simulink model "trajectoryModel"  (Simulink 8.4)
settings: Solver=ode45  StartTime=0.0  StopTime=timeInterval(2)  FixedStep=1e-2  MaxStep=1e-3  RelTol=1e-4  AbsTol=1e-4
values from neighbouring files (symbols this model uses):
  closeRadius = 0.01657    [checkEscapeVelocity.m]
  initialConditions = [x, dx, y, dy]    [checkEscapeVelocity.m]
  mu = Moon_mass / M    (= 0.0121505482564)    [checkEscapeVelocity.m]    (also in computeJacobiCFromRAT.m; velocityPlot_script.m = 0)
  stopRadius = 2    [checkEscapeVelocity.m]
settings Model: Creator=eugene  LastModifiedBy=eugene
settings SolverCC: AutoInsertRateTranBlk=on
settings DataIOCC: SignalLoggingSaveFormat=Dataset
settings OptimizationCC: ExpressionDepthLimit=128  SimCompilerOptimization=On
settings DebuggingCC: UnderspecifiedInitializationDetection=Simplified  MergeDetectMultiDrivingBlocksExec=error  FcnCallInpInsideContextMsg=EnableAllAsError  StateNameClashWarn=none
settings GRTTargetCC: CombineOutputUpdateFcns=on  GRTInterface=off

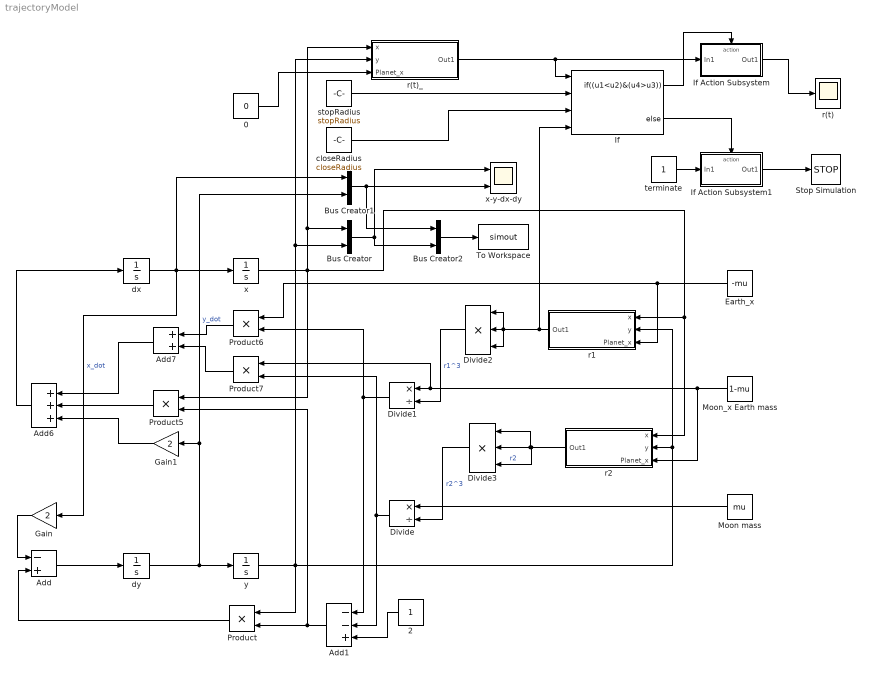
== system trajectoryModel ==
  "0 " : Constant  Value=0
  2 : Constant
  Add : Sum  Inputs=-+
  Add1 : Sum  Inputs=--+
  Add6 : Sum  Inputs=+++
  Add7 : Sum
  Bus Creator : BusCreator  Inputs=2
  Bus Creator1 : BusCreator  Inputs=2
  Bus Creator2 : BusCreator  Inputs=2
  Divide : Product  Inputs=*/
  Divide1 : Product  Inputs=*/
  Divide2 : Product  Inputs=***
  Divide3 : Product  Inputs=***
  Earth_x : Constant  Value=-mu
  Gain : Gain  Gain=2
  Gain1 : Gain  Gain=2
  If : If  NumInputs=4  IfExpression=(u1<u2)&(u4>u3)
  If Action Subsystem : Subsystem  TreatAsAtomicUnit=on
  If Action Subsystem1 : Subsystem  TreatAsAtomicUnit=on
  Moon mass : Constant  Value=mu
  Moon_x Earth mass : Constant  Value=1-mu
  Product{,5..7} (4 alike) : Product
  Stop Simulation : Stop
  To Workspace : ToWorkspace  VariableName=simout  SaveFormat=Timeseries  SampleTime=-1
  closeRadius : Constant  Value=closeRadius
  dx : Integrator  InitialCondition=initialConditions(2)  AbsoluteTolerance=1e-6
  dy : Integrator  InitialCondition=initialConditions(4)  AbsoluteTolerance=1e-6
  r(t) : Scope
      settings: ShowLegends=on  TimeRange=23
  r(t)_ : Subsystem
  r1 : Subsystem
  r2 : Subsystem
  stopRadius : Constant  Value=stopRadius
  terminate : Constant
  x : Integrator  InitialCondition=initialConditions(1)  AbsoluteTolerance=1e-6
  x-y-dx-dy : Scope  NumInputPorts=2
      settings: ShowLegends=on  TimeRange=23  YMin=-5~-5  YMax=5~5  SaveName=ScopeData3
  "y " : Integrator  InitialCondition=initialConditions(3)  AbsoluteTolerance=1e-6
  wires:
  dx/1 -> Bus Creator1/1, Gain/1, x/1  "x_dot"
  dy/1 -> Bus Creator1/2, Gain1/1, "y "/1  "y_dot"
  Earth_x/1 -> Product6/1, r1/3(Planet_x)
  Gain/1 -> Add/1
  Moon_x Earth mass/1 -> Divide1/1, Product7/1, r2/3(Planet_x)
  2/1 -> Add1/3
  Divide/1 -> Product7/2, Add1/2
  Divide1/1 -> Product6/2, Add1/1
  "y "/1 -> Product/1, r2/2(y), r1/2(y), r(t)_/2(y), Bus Creator/2
  Add1/1 -> Product5/2, Product/2
  Product/1 -> Add/2
  Add/1 -> dy/1
  x/1 -> r2/1(x), r1/1(x), Bus Creator/1, r(t)_/1(x), Product5/1
  Divide2/1 -> Divide1/2  "r1^3"
  Divide3/1 -> Divide/2  "r2^3"
  Add6/1 -> dx/1
  Gain1/1 -> Add6/3
  Product5/1 -> Add6/2
  Add7/1 -> Add6/1
  Product6/1 -> Add7/1
  Product7/1 -> Add7/2
  Bus Creator/1 -> Bus Creator2/2, x-y-dx-dy/1
  Bus Creator1/1 -> Bus Creator2/1, x-y-dx-dy/2
  r2/1(Out1) -> Divide3/3, Divide3/1, Divide3/2  "r2"
  Moon mass/1 -> Divide/1
  r(t)_/1(Out1) -> If/1, If Action Subsystem/1(In1)
  "0 "/1 -> r(t)_/3(Planet_x)
  If/1 -> If Action Subsystem/Action
  If/2 -> If Action Subsystem1/Action
  If Action Subsystem/1(Out1) -> r(t)/1
  If Action Subsystem1/1(Out1) -> Stop Simulation/1
  terminate/1 -> If Action Subsystem1/1(In1)
  stopRadius/1 -> If/2
  Bus Creator2/1 -> To Workspace/1
  closeRadius/1 -> If/3
  r1/1(Out1) -> If/4, Divide2/1, Divide2/3, Divide2/2

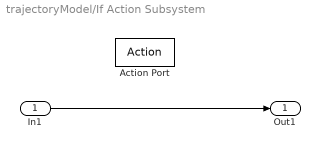
== system trajectoryModel/If Action Subsystem ==
  In1 : Inport
  Action Port : ActionPort  ActionType=then
  Out1 : Outport
  wires:
  In1/1 -> Out1/1

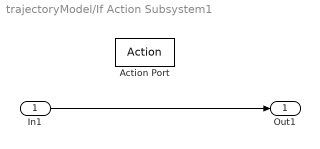
== system trajectoryModel/If Action Subsystem1 ==
  In1 : Inport
  Action Port : ActionPort  ActionType=else
  Out1 : Outport
  wires:
  In1/1 -> Out1/1

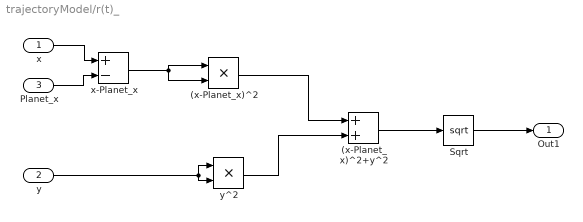
== system trajectoryModel/r(t)_ ==
  x : Inport
  y : Inport  Port=2
  Planet_x : Inport  Port=3
  (x-Planet_x)^2 : Product
  (x-Planet_x)^2+y^2 : Sum
  Sqrt : Sqrt  SaturateOnIntegerOverflow=on
  x-Planet_x : Sum  Inputs=+-
  y^2 : Product
  Out1 : Outport
  wires:
  x/1 -> x-Planet_x/1
  Planet_x/1 -> x-Planet_x/2
  y/1 -> y^2/1, y^2/2
  x-Planet_x/1 -> (x-Planet_x)^2/1, (x-Planet_x)^2/2
  y^2/1 -> (x-Planet_x)^2+y^2/2
  (x-Planet_x)^2/1 -> (x-Planet_x)^2+y^2/1
  (x-Planet_x)^2+y^2/1 -> Sqrt/1
  Sqrt/1 -> Out1/1

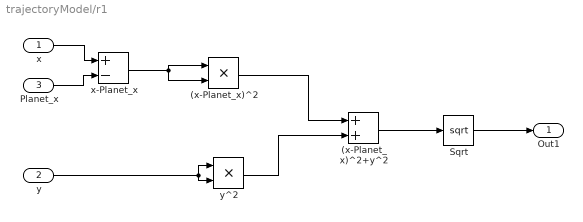
== system trajectoryModel/r1 ==
  x : Inport
  y : Inport  Port=2
  Planet_x : Inport  Port=3
  (x-Planet_x)^2 : Product
  (x-Planet_x)^2+y^2 : Sum
  Sqrt : Sqrt  SaturateOnIntegerOverflow=on
  x-Planet_x : Sum  Inputs=+-
  y^2 : Product
  Out1 : Outport
  wires:
  x/1 -> x-Planet_x/1
  Planet_x/1 -> x-Planet_x/2
  y/1 -> y^2/1, y^2/2
  x-Planet_x/1 -> (x-Planet_x)^2/1, (x-Planet_x)^2/2
  y^2/1 -> (x-Planet_x)^2+y^2/2
  (x-Planet_x)^2/1 -> (x-Planet_x)^2+y^2/1
  (x-Planet_x)^2+y^2/1 -> Sqrt/1
  Sqrt/1 -> Out1/1

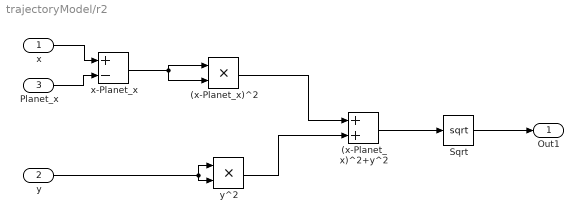
== system trajectoryModel/r2 ==
  x : Inport
  y : Inport  Port=2
  Planet_x : Inport  Port=3
  (x-Planet_x)^2 : Product
  (x-Planet_x)^2+y^2 : Sum
  Sqrt : Sqrt  SaturateOnIntegerOverflow=on
  x-Planet_x : Sum  Inputs=+-
  y^2 : Product
  Out1 : Outport
  wires:
  x/1 -> x-Planet_x/1
  Planet_x/1 -> x-Planet_x/2
  y/1 -> y^2/1, y^2/2
  x-Planet_x/1 -> (x-Planet_x)^2/1, (x-Planet_x)^2/2
  y^2/1 -> (x-Planet_x)^2+y^2/2
  (x-Planet_x)^2/1 -> (x-Planet_x)^2+y^2/1
  (x-Planet_x)^2+y^2/1 -> Sqrt/1
  Sqrt/1 -> Out1/1
